simulink model "Bus8testsystem"  (R2018a)
settings: Solver=FixedStepAuto  StartTime=0.0  StopTime=2.3  RelTol=1e-3  EnableMultiTasking=on
libraries: powerlib x30, powerlib_meascontrol x2
settings Model: Creator=Rodney Tan  LastModifiedBy=pm.deoliveiradejes
settings OptimizationCC: LifeSpan=inf
settings DebuggingCC: SFUnexpectedBacktrackingDiag=warning  SFNoUnconditionalDefaultTransitionDiag=warning
settings CodeAppCC: StateflowObjectComments=on
settings GRTTargetCC: TargetLangStandard=C89/C90 (ANSI)
settings ConfigComp: CovMetricSettings=dw  CovHtmlReporting=on  CovSaveCumulativeToWorkspaceVar=on  CovSaveSingleToWorkspaceVar=on  CovExternalEMLEnable=off
settings SimscapeCC: SimscapeNormalizeSystem=off

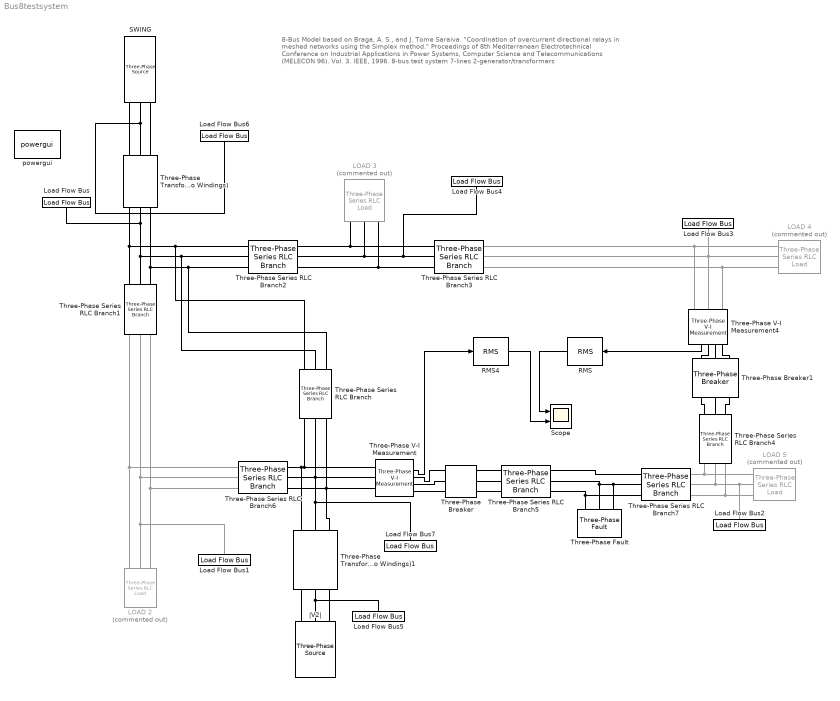
== system Bus8testsystem ==
  note: 8-Bus Model based on
      | Braga, A. S., and J. Tome Saraiva.
      | "Coordination of overcurrent directional relays in meshed networks using the Simplex method."
      | Proceedings of 8th Mediterranean Electrotechnical Conference on Industrial Applications in Power Systems,
      | Computer Science and Telecommunications (MELECON 96). Vol. 3. IEEE, 1996.
      | 8-bus test system 7-lines 2-generator/transformers
  LOAD 2 : powerlib/Elements/Three-Phase Series RLC Load  Commented=on  LConnTagsString=A|B|C  Configuration=Y (grounded)  NominalVoltage=(150000)*1.00894  Vabc=[1e3 1e3 1e3]  Vabcp=[1e3 1e3 1e3]  NominalFrequency=60  UnbalancedPower=off  ActivePower=40e6  InductivePower=20e6  CapacitivePower=0  Pabc=[10e3 9e3 11e3]  QLabc=[100 90 110]  QCabc=[100 90 110]  Pabcp=[10e3 9e3 11e3]  QLabcp=[100 90 110]  QCabcp=[100 90 110]  Measurements=None  LoadType=constant PQ
  LOAD 3 : powerlib/Elements/Three-Phase Series RLC Load  Commented=on  LConnTagsString=A|B|C  Configuration=Y (grounded)  NominalVoltage=(150000)*0.991192  Vabc=[1e3 1e3 1e3]  Vabcp=[1e3 1e3 1e3]  NominalFrequency=60  UnbalancedPower=off  ActivePower=60e6  InductivePower=40e6  CapacitivePower=0  Pabc=[10e3 9e3 11e3]  QLabc=[100 90 110]  QCabc=[100 90 110]  Pabcp=[10e3 9e3 11e3]  QLabcp=[100 90 110]  QCabcp=[100 90 110]  Measurements=None  LoadType=constant PQ
  LOAD 4 : powerlib/Elements/Three-Phase Series RLC Load  Commented=on  LConnTagsString=A|B|C  Configuration=Y (grounded)  NominalVoltage=(150000)*0.99218  Vabc=[1e3 1e3 1e3]  Vabcp=[1e3 1e3 1e3]  NominalFrequency=60  UnbalancedPower=off  ActivePower=70e6  InductivePower=40e6  CapacitivePower=0  Pabc=[10e3 9e3 11e3]  QLabc=[100 90 110]  QCabc=[100 90 110]  Pabcp=[10e3 9e3 11e3]  QLabcp=[100 90 110]  QCabcp=[100 90 110]  Measurements=None  LoadType=constant PQ
  LOAD 5 : powerlib/Elements/Three-Phase Series RLC Load  Commented=on  LConnTagsString=A|B|C  Configuration=Y (grounded)  NominalVoltage=(150000)*1.00274  Vabc=[1e3 1e3 1e3]  Vabcp=[1e3 1e3 1e3]  NominalFrequency=60  UnbalancedPower=off  ActivePower=70e6  InductivePower=50e6  CapacitivePower=0  Pabc=[10e3 9e3 11e3]  QLabc=[100 90 110]  QCabc=[100 90 110]  Pabcp=[10e3 9e3 11e3]  QLabcp=[100 90 110]  QCabcp=[100 90 110]  Measurements=None  LoadType=constant PQ
  Load Flow Bus : powerlib/Measurements/Load Flow Bus  LConnTagsString=a  Phases=single  Connectors=on one side  ID=BUS_1  Vbase=150e3  Vref=1  Vangle=0  VLF=1  VLFb=1  VLFc=1  angleLF=-1.084  angleLFb=0  angleLFc=0
  Load Flow Bus1 : powerlib/Measurements/Load Flow Bus  LConnTagsString=a  Phases=single  Connectors=on one side  ID=BUS_2  Vbase=150e3  Vref=1  Vangle=0  VLF=1.009  VLFb=1  VLFc=1  angleLF=-0.9747  angleLFb=0  angleLFc=0
  Load Flow Bus2 : powerlib/Measurements/Load Flow Bus  LConnTagsString=a  Phases=single  Connectors=on one side  ID=BUS_5  Vbase=150e3  Vref=1  Vangle=0  VLF=1.003  VLFb=1  VLFc=1  angleLF=-1.891  angleLFb=0  angleLFc=0
  Load Flow Bus3 : powerlib/Measurements/Load Flow Bus  LConnTagsString=a  Phases=single  Connectors=on one side  ID=BUS_4  Vbase=150e3  Vref=1  Vangle=0  VLF=0.9922  VLFb=1  VLFc=1  angleLF=-2.378  angleLFb=0  angleLFc=0
  Load Flow Bus4 : powerlib/Measurements/Load Flow Bus  LConnTagsString=a  Phases=single  Connectors=on one side  ID=BUS_3  Vbase=150e3  Vref=1  Vangle=0  VLF=0.9912  VLFb=1  VLFc=1  angleLF=-2.109  angleLFb=0  angleLFc=0
  Load Flow Bus5 : powerlib/Measurements/Load Flow Bus  LConnTagsString=a  Phases=single  Connectors=on one side  ID=BUS_8  Vbase=10e3  Vref=1  Vangle=0  VLF=1.074  VLFb=1  VLFc=1  angleLF=1.383  angleLFb=0  angleLFc=0
  Load Flow Bus6 : powerlib/Measurements/Load Flow Bus  LConnTagsString=a  Phases=single  Connectors=on one side  ID=BUS_7  Vbase=10e3  Vref=1  Vangle=0  VLF=1  VLFb=1  VLFc=1  angleLF=0  angleLFb=0  angleLFc=0
  Load Flow Bus7 : powerlib/Measurements/Load Flow Bus  LConnTagsString=a  Phases=single  Connectors=on one side  ID=BUS_6  Vbase=150e3  Vref=1  Vangle=0  VLF=1.025  VLFb=1  VLFc=1  angleLF=-0.6996  angleLFb=0  angleLFc=0
  RMS : powerlib_meascontrol/Measurements/RMS  TrueRMS=on  Freq=60  RMSInit=120  Ts=0
  RMS4 : powerlib_meascontrol/Measurements/RMS  TrueRMS=on  Freq=60  RMSInit=120  Ts=0
  SWING : powerlib/Electrical Sources/Three-Phase Source  InternalConnection=Yg  VoltagePhases=off  Voltage=10000  PhaseAngle=0  Voltage_phases=[25e3 25e3 25e3]/sqrt(3)  PhaseAngles_phases=[0 -120 +120]  Frequency=60  NonIdealSource=on  SpecifyImpedance=off  Resistance=00  Inductance=.15*10*10/150/377  ShortCircuitLevel=100e6  BaseVoltage=10000  XRratio=7  BusType=swing  Pref=10e3  Qref=0  Prefabc=[10e3, 10e3, 10e3]  Qrefabc=[0, 0, 0]  Qmin=-inf  Qmax=inf
  Scope : Scope  NumInputPorts=2
  Three-Phase Series RLC Branch : powerlib/Elements/Three-Phase Series RLC Branch  LConnTagsString=A|B|C  RConnTagsString=A|B|C  BranchType=RL  Resistance=0.005*100  Inductance=100*0.05/377  Capacitance=1e-6  Measurements=None
  Three-Phase Series RLC Branch1 : powerlib/Elements/Three-Phase Series RLC Branch  LConnTagsString=A|B|C  RConnTagsString=A|B|C  BranchType=RL  Resistance=0.004*100  Inductance=(100*0.05)/377  Capacitance=1e-6  Measurements=None
  Three-Phase Series RLC Branch2 : powerlib/Elements/Three-Phase Series RLC Branch  LConnTagsString=A|B|C  RConnTagsString=A|B|C  BranchType=RL  Resistance=0.0057*70  Inductance=70*0.0714/377  Capacitance=1e-6  Measurements=None
  Three-Phase Series RLC Branch3 : powerlib/Elements/Three-Phase Series RLC Branch  LConnTagsString=A|B|C  RConnTagsString=A|B|C  BranchType=RL  Resistance=0.005*80  Inductance=80*0.0563/377  Capacitance=1e-6  Measurements=None
  Three-Phase Series RLC Branch4 : powerlib/Elements/Three-Phase Series RLC Branch  LConnTagsString=A|B|C  RConnTagsString=A|B|C  BranchType=RL  Resistance=0.005*100  Inductance=100*0.045/377  Capacitance=1e-6  Measurements=None
  Three-Phase Series RLC Branch5 : powerlib/Elements/Three-Phase Series RLC Branch  LConnTagsString=A|B|C  RConnTagsString=A|B|C  BranchType=RL  Resistance=0.0045*110*(1-.9209)  Inductance=110*0.0409*(1-.9209)/377  Capacitance=1e-6  Measurements=None
  Three-Phase Series RLC Branch6 : powerlib/Elements/Three-Phase Series RLC Branch  LConnTagsString=A|B|C  RConnTagsString=A|B|C  BranchType=RL  Resistance=0.0044*90  Inductance=90*0.05/377  Capacitance=1e-6  Measurements=None
  Three-Phase Series RLC Branch7 : powerlib/Elements/Three-Phase Series RLC Branch  LConnTagsString=A|B|C  RConnTagsString=A|B|C  BranchType=RL  Resistance=0.0045*110*.9209  Inductance=110*0.0409*.9209/377  Capacitance=1e-6  Measurements=None
  Three-Phase V-I Measurement : powerlib/Measurements/Three-Phase V-I Measurement  VoltageMeasurement=phase-to-ground  SetLabelV=off  LabelV=Vabc  Vpu=off  VpuLL=off  CurrentMeasurement=yes  SetLabelI=off  LabelI=Iabc  Ipu=off  Pbase=100e6  Vbase=500e3  OutputType=Complex  PhasorSimulation=off  PSBequivalent=0
  Three-Phase V-I Measurement4 : powerlib/Measurements/Three-Phase V-I Measurement  VoltageMeasurement=phase-to-ground  SetLabelV=off  LabelV=Vabc  Vpu=off  VpuLL=off  CurrentMeasurement=yes  SetLabelI=off  LabelI=Iabc  Ipu=off  Pbase=100e6  Vbase=500e3  OutputType=Complex  PhasorSimulation=off  PSBequivalent=0
  Three-Phase Breaker : powerlib/Elements/Three-Phase Breaker  InitialState=closed  SwitchA=on  SwitchB=on  SwitchC=on  SwitchTimes=[0.99 10]  External=off  BreakerResistance=0.00000001  SnubberResistance=1e6  SnubberCapacitance=inf  Measurements=None
  Three-Phase Breaker1 : powerlib/Elements/Three-Phase Breaker  InitialState=closed  SwitchA=on  SwitchB=on  SwitchC=on  SwitchTimes=[2.21 10]  External=off  BreakerResistance=0.00000001  SnubberResistance=1e6  SnubberCapacitance=inf  Measurements=None
  Three-Phase Fault : powerlib/Elements/Three-Phase Fault  InitialStates=0  FaultA=on  FaultB=on  FaultC=on  GroundFault=on  SwitchTimes="[1/60  60/60]"  External=off  SwitchStatus=NaN  FaultResistance=0.0000001  GroundResistance=0.0000001  SnubberResistance=0.0000001  SnubberCapacitance=inf  Measurements=None
  Three-Phase Transformer Inductance Matrix Type (Two Windings) : powerlib/Elements/Three-Phase Transformer Inductance Matrix Type (Two Windings)  CoreType=Three single-phase cores  Winding1Connection=Yg  Winding2Connection=Yg  AutoTransformer=off  Measurements=None  NominalPower=[150e6, 60]  VLLnom=[150000, 10000]  WindingResistances=[0.0000000001, 0.00000000001]  NoLoadIexcPos=1  NoLoadPlossPos=10  ShortCircuitReactancePos=0.04  ShortCircuitReactancePosAuto=0.06  NoLoadIexcZero=100  NoLoadPlossZero=1500  ShortCircuitReactanceZero=0.03  ShortCircuitReactanceZeroAuto=0.03
      settings: SourceProductName=Simscape Power Systems  SourceProductBaseCode=PS
  Three-Phase Transformer Inductance Matrix Type (Two Windings)1 : powerlib/Elements/Three-Phase Transformer Inductance Matrix Type (Two Windings)  CoreType=Three single-phase cores  Winding1Connection=Yg  Winding2Connection=Yg  AutoTransformer=off  Measurements=None  NominalPower=[150e6, 60]  VLLnom=[150000, 10000]  WindingResistances=[0.0000000001, 0.00000000001]  NoLoadIexcPos=1  NoLoadPlossPos=10  ShortCircuitReactancePos=0.04  ShortCircuitReactancePosAuto=0.06  NoLoadIexcZero=100  NoLoadPlossZero=1500  ShortCircuitReactanceZero=0.03  ShortCircuitReactanceZeroAuto=0.03
      settings: SourceProductName=Simscape Power Systems  SourceProductBaseCode=PS
  powergui : powerlib/powergui  Priority=1  SimulationMode=Discrete  SampleTime=50e-6  frequency=60  Iterations=50  frequencyindice=0  Pbase=100e6  ErrMax=0.0001  UnitsV=kV  UnitsW=MW  buscounter=0  FunctionMessages=off  echomessages=off  EnableUseOfTLC=off  CurrentSourceSwitches=off  DisableSnubberDevices=off  DisableRonSwitches=off  DisableVfSwitches=off  DisplayEquations=off  SolverType=Tustin/Backward Euler (TBE)  Interpol=off  ExternalGateDelay=off  methode=off  Ts=100  x0status=blocks  SPID=off  SwTol=0  HookPort=off  RestoreLinks=warning  ResistiveCurrentMeasurement=off  Frange=[0:2:500]  Ylog=off  Xlog=on  ShowGrid=off  save=off  variable=ZData  structure=0  ZoomFFT=off  StartTime=0.0  cycles=1  DisplayStyle=1  fundamental=60  FreqAxis=off  MaxFrequency=1000  frequencyindicesteady=0 Hz  RmsSteady=2  display=off
  |V2| : powerlib/Electrical Sources/Three-Phase Source  InternalConnection=Yg  VoltagePhases=off  Voltage=10000  PhaseAngle=0  Voltage_phases=[25e3 25e3 25e3]/sqrt(3)  PhaseAngles_phases=[0 -120 +120]  Frequency=60  NonIdealSource=on  SpecifyImpedance=off  Resistance=0  Inductance=.15*10*10/150/377  ShortCircuitLevel=100e6  BaseVoltage=10000  XRratio=7  BusType=PQ  Pref=150e6  Qref=0  Prefabc=[10e3, 10e3, 10e3]  Qrefabc=[0, 0, 0]  Qmin=-200e6  Qmax=200e6
  wires:
  Three-Phase V-I Measurement/2 -> RMS4/1
  RMS4/1 -> Scope/2
  RMS/1 -> Scope/1
  Three-Phase V-I Measurement4/2 -> RMS/1
  connections:
  Three-Phase Transformer Inductance Matrix Type (Two Windings)/LConn2 -- Load Flow Bus/LConn1 -- Three-Phase Series RLC Branch/LConn2 -- Three-Phase Series RLC Branch2/LConn2 -- Three-Phase Series RLC Branch1/LConn2
  Three-Phase Transformer Inductance Matrix Type (Two Windings)/LConn1 -- Three-Phase Series RLC Branch/LConn1 -- Three-Phase Series RLC Branch2/LConn1 -- Three-Phase Series RLC Branch1/LConn1
  LOAD 2/LConn2 -- Load Flow Bus1/LConn1 -- Three-Phase Series RLC Branch6/LConn2 -- Three-Phase Series RLC Branch1/RConn2
  LOAD 2/LConn3 -- Three-Phase Series RLC Branch6/LConn3 -- Three-Phase Series RLC Branch1/RConn3
  Three-Phase Series RLC Branch1/LConn3 -- Three-Phase Series RLC Branch/LConn3 -- Three-Phase Series RLC Branch2/LConn3 -- Three-Phase Transformer Inductance Matrix Type (Two Windings)/LConn3
  Three-Phase Series RLC Branch2/RConn1 -- Three-Phase Series RLC Branch3/LConn1 -- LOAD 3/LConn1
  Three-Phase Series RLC Branch2/RConn2 -- Load Flow Bus4/LConn1 -- Three-Phase Series RLC Branch3/LConn2 -- LOAD 3/LConn2
  Three-Phase Series RLC Branch2/RConn3 -- Three-Phase Series RLC Branch3/LConn3 -- LOAD 3/LConn3
  LOAD 2/LConn1 -- Three-Phase Series RLC Branch6/LConn1 -- Three-Phase Series RLC Branch1/RConn1
  Three-Phase Series RLC Branch4/LConn1 -- Three-Phase Breaker1/LConn1
  Three-Phase Series RLC Branch4/LConn2 -- Three-Phase Breaker1/LConn2
  Three-Phase Series RLC Branch4/LConn3 -- Three-Phase Breaker1/LConn3
  SWING/RConn1 -- Three-Phase Transformer Inductance Matrix Type (Two Windings)/RConn1
  Three-Phase Transformer Inductance Matrix Type (Two Windings)/RConn2 -- Load Flow Bus6/LConn1 -- SWING/RConn2
  Three-Phase Transformer Inductance Matrix Type (Two Windings)/RConn3 -- SWING/RConn3
  Three-Phase Transformer Inductance Matrix Type (Two Windings)1/RConn2 -- Load Flow Bus5/LConn1 -- |V2|/RConn2
  Three-Phase Transformer Inductance Matrix Type (Two Windings)1/RConn1 -- |V2|/RConn1
  |V2|/RConn3 -- Three-Phase Transformer Inductance Matrix Type (Two Windings)1/RConn3
  Three-Phase V-I Measurement/LConn2 -- Load Flow Bus7/LConn1 -- Three-Phase Transformer Inductance Matrix Type (Two Windings)1/LConn2 -- Three-Phase Series RLC Branch/RConn2 -- Three-Phase Series RLC Branch6/RConn2
  Three-Phase V-I Measurement/LConn1 -- Three-Phase Transformer Inductance Matrix Type (Two Windings)1/LConn1 -- Three-Phase Series RLC Branch6/RConn1 -- Three-Phase Series RLC Branch/RConn1
  Three-Phase V-I Measurement/LConn3 -- Three-Phase Transformer Inductance Matrix Type (Two Windings)1/LConn3 -- Three-Phase Series RLC Branch/RConn3 -- Three-Phase Series RLC Branch6/RConn3
  Three-Phase Breaker/RConn2 -- Three-Phase Series RLC Branch5/LConn2
  Three-Phase Series RLC Branch5/RConn2 -- Three-Phase Fault/LConn2 -- Three-Phase Fault/LConn1 -- Three-Phase Series RLC Branch7/LConn2
  Three-Phase Breaker/RConn3 -- Three-Phase Series RLC Branch5/LConn3
  Three-Phase Breaker/RConn1 -- Three-Phase Series RLC Branch5/LConn1
  Three-Phase Series RLC Branch5/RConn3 -- Three-Phase Fault/LConn3 -- Three-Phase Series RLC Branch7/LConn3
  Three-Phase Series RLC Branch5/RConn1 -- Three-Phase Series RLC Branch7/LConn1
  LOAD 5/LConn2 -- Load Flow Bus2/LConn1 -- Three-Phase Series RLC Branch4/RConn2 -- Three-Phase Series RLC Branch7/RConn2
  LOAD 5/LConn1 -- Three-Phase Series RLC Branch4/RConn1 -- Three-Phase Series RLC Branch7/RConn1
  LOAD 5/LConn3 -- Three-Phase Series RLC Branch4/RConn3 -- Three-Phase Series RLC Branch7/RConn3
  Three-Phase V-I Measurement/RConn3 -- Three-Phase Breaker/LConn3
  Three-Phase V-I Measurement/RConn2 -- Three-Phase Breaker/LConn2
  Three-Phase V-I Measurement/RConn1 -- Three-Phase Breaker/LConn1
  Three-Phase V-I Measurement4/RConn2 -- Three-Phase Breaker1/RConn2
  Three-Phase V-I Measurement4/RConn1 -- Three-Phase Breaker1/RConn1
  Three-Phase V-I Measurement4/RConn3 -- Three-Phase Breaker1/RConn3
  LOAD 4/LConn2 -- Load Flow Bus3/LConn1 -- Three-Phase V-I Measurement4/LConn2 -- Three-Phase Series RLC Branch3/RConn2
  LOAD 4/LConn3 -- Three-Phase V-I Measurement4/LConn3 -- Three-Phase Series RLC Branch3/RConn3
  LOAD 4/LConn1 -- Three-Phase V-I Measurement4/LConn1 -- Three-Phase Series RLC Branch3/RConn1
